simulink model "Problem8"  (R2020a)
settings: Solver=VariableStepAuto  StartTime=0.0  StopTime=10.0  RelTol=1e-3
settings Model: Creator=tanu  LastModifiedBy=tanu

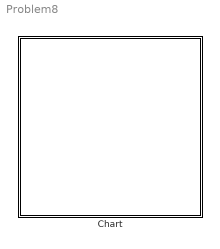
== system Problem8 ==
  Chart : Stateflow chart  TreatAsAtomicUnit=on

== stateflow chart Problem8/Chart ==
  state State1
  (default) -> State1
